simulink model "model"  (R2018b)
settings: Solver=ode4  StartTime=0.0  StopTime=10.0  FixedStep=1e-2  RelTol=1
values from neighbouring files (symbols this model uses):
  A = total_intrest    (= 1.04)    [Capitalization.m]    (also in DiscretSystem.m = lamda(i); DiscreteVsContinues.m = expm(h*A_c))
  B = 0    [Capitalization.m]    (also in DiscretSystem.m; DiscreteVsContinues.m = double(int(expm(z*A_c)*B_c,z,0,h)))
  C = 1    [Capitalization.m]    (also in DiscretSystem.m; DiscreteVsContinues.m = C_c)
  D = 0    [Capitalization.m]    (also in DiscretSystem.m; DiscreteVsContinues.m = D_c)
  h = cap_rate    [Capitalization.m]    (also in DiscretSystem.m = 1; DiscreteVsContinues.m = 1)
  Start = 10000    [Capitalization.m]    (also in DiscretSystem.m = 10; DiscreteVsContinues.m = 5)
settings Model: Creator=bion  LastModifiedBy=bion

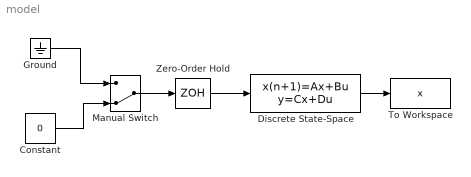
== system model ==
  Constant : Constant  Value=0  SampleTime=h
  Discrete State-Space : DiscreteStateSpace  A=A  B=B  C=C  D=D  InitialCondition=Start  SampleTime=h
  Ground : Ground
  Manual Switch : ManualSwitch  CurrentSetting=0
  To Workspace : ToWorkspace  VariableName=x  SampleTime=1e-2
  Zero-Order Hold : ZeroOrderHold  SampleTime=h
  wires:
  Zero-Order Hold/1 -> Discrete State-Space/1
  Discrete State-Space/1 -> To Workspace/1
  Manual Switch/1 -> Zero-Order Hold/1
  Constant/1 -> Manual Switch/2
  Ground/1 -> Manual Switch/1
